simulink model "d_kundur1"  (Simulink 5.1)
settings: Solver=ode45  StartTime=0.0  StopTime=10.0  RelTol=1e-3
libraries: fm_lib x15
settings Model: Creator=fmilano  LastModifiedBy=fmilano  ExtModeAutoUpdateStatusClock=off  SignalLoggingName=logsout  BooleanDataType=on  RTWOptions="-aEnforceIntegerDowncast=1 -aFoldNonRolledExpr=1 -aInlineInvariantSignals=1 -aInlineParameters=0 -aLocalBlockOutputs=1 -aRollThreshold=5 -aZeroInternalMemoryAtStartup=1 -aZeroExternalMemoryAtStartup=1 -aInitFltsAndDblsToZero=1 -aForceBlockIOInitOptimize=0 -aGenerateReport=0 -aGenCodeOnly=0 -aRTWVerbose=1 -aIncludeHyperlinkInReport=0 -aLaunchReport=0 -aGenerateTraceInfo=0  -aForceParamTrailComments=0 -aGenerateComments=1 -aIgnoreCustomStorageClasses=1 -aIncHierarchyInIds=0 -aMaxRTWIdLen=31 -aShowEliminatedStatements=0 -aIncDataTypeInIds=0 -aInsertBlockDesc=0 -aIgnoreTestpoints=0 -aSimulinkBlockComments=1 -aInlinedPrmAccess=\"Literals\"  -aSuppressErrorStatus=0 -aModelReferenceCompliant=1 -aParenthesesLevel=\"Nominal\" -aModelStepFunctionPrototypeControlCompliant=0 -aPortableWordSizes=0 -aParMdlRefBuildCompliant=1 -aSupportNonInlinedSFcns=1 -aSupportContinuousTime=1 -aSupportComplex=1 -aSupportNonFinite=1 -aSupportAbsoluteTime=1 -aMultiwordLength=2048 -aTargetPreCompLibLocation=\"\" -aTargetLibSuffix=\"\" -aTargetFunctionLibrary=\"ANSI_C\" -aTargetFcnLib=\"ansi_tfl_tmw.mat\" -aMultiInstanceERTCode=0 -aLogVarNameModifier=\"rt_\" -aERTFirstTimeCompliant=0 -aIsPILTarget=0 -aCombineOutputUpdateFcns=0 -aGenerateASAP2=0 -aGenerateClassInterface=0 -aGenerateTestInterfaces=0 -aGenerateSampleERTMain=0 -aGenerateFullHeader=1 -aUtilityFuncGeneration=\"Auto\" -aIncludeFileDelimiter=\"Auto\" -aIncludeMdlTerminateFcn=1 -aPurelyIntegerCode=0 -aAutosarCompliant=0 -aERTCustomFileBanners=0 -aRTWCAPIStates=0 -aRTWCAPIParams=0 -aRTWCAPISignals=0 -aMatFileLogging=1 -aCompOptLevelCompliant=0 -aCPPClassGenCompliant=0 -aExtModeIntrfLevel=\"Level1\" -aExtModeMexFile=\"ext_comm\" -aExtModeTransport=0 -aExtModeStaticAllocSize=1000000 -aExtModeTesting=0 -aExtModeStaticAlloc=0 -aExtMode=0 -aERTMultiwordLength=256 -aERTMultiwordTypeDef=\"System defined\"  -aGenerateTraceInfo=0 -aGenerateTraceInfo=0 -aGenerateTraceInfo=0 -aGenerateTraceInfo=0 -aPrefixModelToSubsysFcnNames=1"

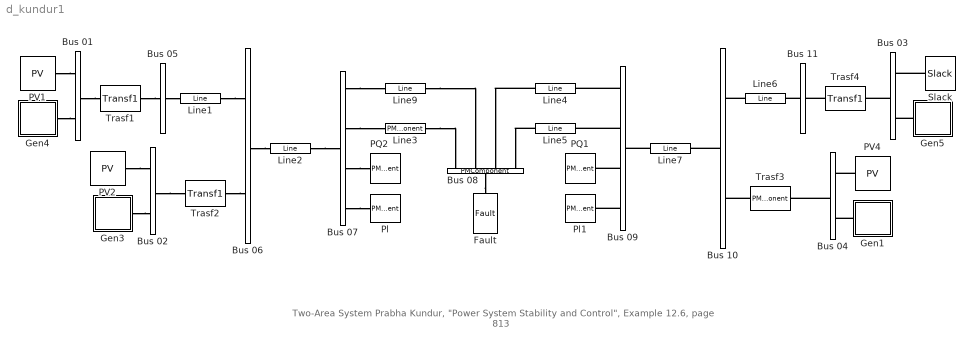
== system d_kundur1 ==
  note: Two-Area System
      | Prabha Kundur, "Power System Stability and Control", Example 12.6, page 813
  Bus 01 : PMComponent  Tag=PSATblock  Description=Connection  PhysicalDomain=psatdomain  LeftPortType=p1  RightPortType=p1  LConnTagsString=__newl0|__newl1  RConnTagsString=__newr0  mask(Bus){in=2, out=1, p2q=20, p3_4q=[1.03   0.3229], p5q=1, p6q=1}
      mask prompts: in "Number of inputs:"; out "Number of outputs:"; p2q "Voltage Rating [kV]"; p3_4q "Voltage initial guess [p.u.  rad]"; p5q "Area number"; p6q "Region number"
      mask help: Bus block.
      mask init:
      | fm_inout
      mask CallbackString: ||||fm_block|
      mask Display: plot([0 1 1 0 0],[0 0 1 1 0])
  Bus 02 : PMComponent  Tag=PSATblock  Description=Connection  PhysicalDomain=psatdomain  LeftPortType=p1  RightPortType=p1  LConnTagsString=__newl0|__newl1  RConnTagsString=__newr0  mask(Bus){in=2, out=1, p2q=20, p3_4q=[1.01   0.1536], p5q=1, p6q=1}
      mask prompts: in "Number of inputs:"; out "Number of outputs:"; p2q "Voltage Rating [kV]"; p3_4q "Voltage initial guess [p.u.  rad]"; p5q "Area number"; p6q "Region number"
      mask help: Bus block.
      mask init:
      | fm_inout
      mask CallbackString: ||||fm_block|
      mask Display: plot([0 1 1 0 0],[0 0 1 1 0])
  Bus 03 : PMComponent  Tag=PSATblock  Description=Connection  Orientation=left  PhysicalDomain=psatdomain  LeftPortType=p1  RightPortType=p1  LConnTagsString=__newl0|__newl1  RConnTagsString=__newr0  mask(Bus){in=2, out=1, p2q=20, p3_4q=[1.03  -0.1187], p5q=2, p6q=1}
      mask prompts: in "Number of inputs:"; out "Number of outputs:"; p2q "Voltage Rating [kV]"; p3_4q "Voltage initial guess [p.u.  rad]"; p5q "Area number"; p6q "Region number"
      mask help: Bus block.
      mask init:
      | fm_inout
      mask CallbackString: ||||fm_block|
      mask Display: plot([0 1 1 0 0],[0 0 1 1 0])
  Bus 04 : PMComponent  Tag=PSATblock  Description=Connection  Orientation=left  PhysicalDomain=psatdomain  LeftPortType=p1  RightPortType=p1  LConnTagsString=__newl0|__newl1  RConnTagsString=__newr0  mask(Bus){in=2, out=1, p2q=20, p3_4q=[1.01   -0.295], p5q=2, p6q=1}
      mask prompts: in "Number of inputs:"; out "Number of outputs:"; p2q "Voltage Rating [kV]"; p3_4q "Voltage initial guess [p.u.  rad]"; p5q "Area number"; p6q "Region number"
      mask help: Bus block.
      mask init:
      | fm_inout
      mask CallbackString: ||||fm_block|
      mask Display: plot([0 1 1 0 0],[0 0 1 1 0])
  Bus 05 : PMComponent  Tag=PSATblock  Description=Connection  PhysicalDomain=psatdomain  LeftPortType=p1  RightPortType=p1  LConnTagsString=__newl0  RConnTagsString=__newr0  mask(Bus){in=1, out=1, p2q=230, p3_4q=[1.01   0.2112], p5q=1, p6q=1}
      mask prompts: in "Number of inputs:"; out "Number of outputs:"; p2q "Voltage Rating [kV]"; p3_4q "Voltage initial guess [p.u.  rad]"; p5q "Area number"; p6q "Region number"
      mask help: Bus block.
      mask init:
      | fm_inout
      mask CallbackString: ||||fm_block|
      mask Display: plot([0 1 1 0 0],[0 0 1 1 0])
  Bus 06 : PMComponent  Tag=PSATblock  Description=Connection  PhysicalDomain=psatdomain  LeftPortType=p1  RightPortType=p1  LConnTagsString=__newl0|__newl1  RConnTagsString=__newr0  mask(Bus){in=2, out=1, p2q=230, p3_4q=[0.9876   0.03665], p5q=1, p6q=1}
      mask prompts: in "Number of inputs:"; out "Number of outputs:"; p2q "Voltage Rating [kV]"; p3_4q "Voltage initial guess [p.u.  rad]"; p5q "Area number"; p6q "Region number"
      mask help: Bus block.
      mask init:
      | fm_inout
      mask CallbackString: ||||fm_block|
      mask Display: plot([0 1 1 0 0],[0 0 1 1 0])
  Bus 07 : PMComponent  Tag=PSATblock  Description=Connection  PhysicalDomain=psatdomain  LeftPortType=p1  RightPortType=p1  LConnTagsString=__newl0  RConnTagsString=__newr0|__newr1|__newr2|__newr3  mask(Bus){in=1, out=4, p2q=230, p3_4q=[1   -0.1065], p5q=1, p6q=1}
      mask prompts: in "Number of inputs:"; out "Number of outputs:"; p2q "Voltage Rating [kV]"; p3_4q "Voltage initial guess [p.u.  rad]"; p5q "Area number"; p6q "Region number"
      mask help: Bus block.
      mask init:
      | fm_inout
      mask CallbackString: ||||fm_block|
      mask Display: plot([0 1 1 0 0],[0 0 1 1 0])
  Bus 08 : PMComponent  Tag=PSATblock  Description=Connection  Orientation=down  PhysicalDomain=psatdomain  LeftPortType=p1  RightPortType=p1  LConnTagsString=__newl0|__newl1|__newl2|__newl3  RConnTagsString=__newr0  mask(Bus){in=4, out=1, p2q=230, p3_4q=[1.0   -0.3368], p5q=3, p6q=1}
      mask prompts: in "Number of inputs:"; out "Number of outputs:"; p2q "Voltage Rating [kV]"; p3_4q "Voltage initial guess [p.u.  rad]"; p5q "Area number"; p6q "Region number"
      mask help: Bus block.
      mask init:
      | fm_inout
      mask CallbackString: ||||fm_block|
      mask Display: plot([0 1 1 0 0],[0 0 1 1 0])
  Bus 09 : PMComponent  Tag=PSATblock  Description=Connection  Orientation=left  PhysicalDomain=psatdomain  LeftPortType=p1  RightPortType=p1  LConnTagsString=__newl0  RConnTagsString=__newr0|__newr1|__newr2|__newr3  mask(Bus){in=1, out=4, p2q=230, p3_4q=[0.9899   -0.555], p5q=2, p6q=1}
      mask prompts: in "Number of inputs:"; out "Number of outputs:"; p2q "Voltage Rating [kV]"; p3_4q "Voltage initial guess [p.u.  rad]"; p5q "Area number"; p6q "Region number"
      mask help: Bus block.
      mask init:
      | fm_inout
      mask CallbackString: ||||fm_block|
      mask Display: plot([0 1 1 0 0],[0 0 1 1 0])
  Bus 10 : PMComponent  Tag=PSATblock  Description=Connection  Orientation=left  PhysicalDomain=psatdomain  LeftPortType=p1  RightPortType=p1  LConnTagsString=__newl0|__newl1  RConnTagsString=__newr0  mask(Bus){in=2, out=1, p2q=230, p3_4q=[0.9938   -0.4119], p5q=2, p6q=1}
      mask prompts: in "Number of inputs:"; out "Number of outputs:"; p2q "Voltage Rating [kV]"; p3_4q "Voltage initial guess [p.u.  rad]"; p5q "Area number"; p6q "Region number"
      mask help: Bus block.
      mask init:
      | fm_inout
      mask CallbackString: ||||fm_block|
      mask Display: plot([0 1 1 0 0],[0 0 1 1 0])
  Bus 11 : PMComponent  Tag=PSATblock  Description=Connection  Orientation=left  PhysicalDomain=psatdomain  LeftPortType=p1  RightPortType=p1  LConnTagsString=__newl0  RConnTagsString=__newr0  mask(Bus){in=1, out=1, p2q=230, p3_4q=[1.013   -0.233900], p5q=2, p6q=1}
      mask prompts: in "Number of inputs:"; out "Number of outputs:"; p2q "Voltage Rating [kV]"; p3_4q "Voltage initial guess [p.u.  rad]"; p5q "Area number"; p6q "Region number"
      mask help: Bus block.
      mask init:
      | fm_inout
      mask CallbackString: ||||fm_block|
      mask Display: plot([0 1 1 0 0],[0 0 1 1 0])
  Fault : fm_lib/Faults &  Breakers/Fault  Tag=PSATblock  Description=Faults & Breakers  Orientation=down  PhysicalDomain=psatdomain  SubClassName=unknown  LeftPortType=p1  RightPortType=p1  LConnTagsString=__newl0  p2_3_4q="[100  230  60]"  p5q=1  p6q=1.050  p7q=0  p8q=1e-5
  Gen1 : Subsystem  Tag=PSATblock  Description=Machines  Orientation=left  mask(Syn){p2_3_4q=[900  20  60], p5q=6, p7_6q=[0.0025  0.2], p8_9_10q=[1.80  0.30  0.25], p11_12q=[8.00  0.03], p13_14_15q=[1.70  0.55  0.25], p16_17q=[0.4  0.05], p18_19q=[12.35  0.00], p20_21q=[0.00  0.00], p22_23q=[1.00  1.00], p24q=0.0, p25_26q=[0 0], in=0, p27q=1, p28q=on}
      mask prompts: p2_3_4q "Power, voltage and frequency ratings [MVA, kV, Hz]"; p5q "Machine Dynamic Order"; p7_6q "resistance ra and leakage reactance xl [p.u. p.u.]"; p8_9_10q "d-axis reactances Xd, X'd X"d [p.u.,p.u.,p.u.]"; p11_12q "d-axis open circuit time constants T'd0 and T"d0 [s, s]"; p13_14_15q "q-axis reactances Xq, X'q, X"q [p.u.  p.u.  p.u.]"; p16_17q "q-axis open circuit time constants T'q0 and T"q0 [s s]"; p18_19q "Inertia (M = 2H) and Damping [s, p.u.]"; p20_21q "Speed and active power additional signals Kw and Kp [p.u., p.u.]"; p22_23q "Percentage of active and reactive powers at bus [p.u. p.u.]"; p24q "d-axis additional circuit leakage time constant Taa [s]"; p25_26q "Saturation coefficients S(1.0) and S(1.2)"; in "Number of input signals"; p27q "COI number"; p28q "Connected"
      mask help: This block defines a fourth order synchronous machine.
      mask init:
      | fm_inout
      | [x,y] = fm_draw('circle');
      | [xg,yg] = fm_draw('G');
      | [xs,ys] = fm_draw('sinus');
      mask StyleString: edit,popup(8|6|5.3|5.2|5.1|4|3|2),edit,edit,edit,edit,edit,edit,edit,edit,edit,edit,popup(0|1|2),edit,checkbox
      mask CallbackString: |fm_block|||||||||||||fm_block
      mask Display:
      | plot(x+1.4,y,0.12*xs+1,0.15*ys-0.6)
      | color('blue')
      | plot(1.4+0.45*xg,0.3+0.45*yg)
  Gen3 : Subsystem  Tag=PSATblock  Description=Machines  mask(Syn){p2_3_4q=[900  20  60], p5q=6, p7_6q=[0.0025  0.2], p8_9_10q=[1.80  0.30  0.25], p11_12q=[8.00  0.03], p13_14_15q=[1.70  0.55  0.25], p16_17q=[0.4  0.05], p18_19q=[13.00  0.00], p20_21q=[0.00  0.00], p22_23q=[1.00  1.00], p24q=0.0, p25_26q=[0 0], in=0, p27q=1, p28q=on}
      mask prompts: p2_3_4q "Power, voltage and frequency ratings [MVA, kV, Hz]"; p5q "Machine Dynamic Order"; p7_6q "resistance ra and leakage reactance xl [p.u. p.u.]"; p8_9_10q "d-axis reactances Xd, X'd X"d [p.u.,p.u.,p.u.]"; p11_12q "d-axis open circuit time constants T'd0 and T"d0 [s, s]"; p13_14_15q "q-axis reactances Xq, X'q, X"q [p.u.  p.u.  p.u.]"; p16_17q "q-axis open circuit time constants T'q0 and T"q0 [s s]"; p18_19q "Inertia (M = 2H) and Damping [s, p.u.]"; p20_21q "Speed and active power additional signals Kw and Kp [p.u., p.u.]"; p22_23q "Percentage of active and reactive powers at bus [p.u. p.u.]"; p24q "d-axis additional circuit leakage time constant Taa [s]"; p25_26q "Saturation coefficients S(1.0) and S(1.2)"; in "Number of input signals"; p27q "COI number"; p28q "Connected"
      mask help: This block defines a fourth order synchronous machine.
      mask init:
      | fm_inout
      | [x,y] = fm_draw('circle');
      | [xg,yg] = fm_draw('G');
      | [xs,ys] = fm_draw('sinus');
      mask StyleString: edit,popup(8|6|5.3|5.2|5.1|4|3|2),edit,edit,edit,edit,edit,edit,edit,edit,edit,edit,popup(0|1|2),edit,checkbox
      mask CallbackString: |fm_block|||||||||||||fm_block
      mask Display:
      | plot(x+1.4,y,0.12*xs+1,0.15*ys-0.6)
      | color('blue')
      | plot(1.4+0.45*xg,0.3+0.45*yg)
  Gen4 : Subsystem  Tag=PSATblock  Description=Machines  mask(Syn){p2_3_4q=[900  20  60], p5q=6, p7_6q=[0.0025  0.2], p8_9_10q=[1.80  0.30  0.25], p11_12q=[8.00  0.03], p13_14_15q=[1.70  0.55  0.25], p16_17q=[0.4  0.05], p18_19q=[13.00  0.00], p20_21q=[0.00  0.00], p22_23q=[1.00  1.00], p24q=0.002, p25_26q=[0 0], in=0, p27q=1, p28q=on}
      mask prompts: p2_3_4q "Power, voltage and frequency ratings [MVA, kV, Hz]"; p5q "Machine Dynamic Order"; p7_6q "resistance ra and leakage reactance xl [p.u. p.u.]"; p8_9_10q "d-axis reactances Xd, X'd X"d [p.u.,p.u.,p.u.]"; p11_12q "d-axis open circuit time constants T'd0 and T"d0 [s, s]"; p13_14_15q "q-axis reactances Xq, X'q, X"q [p.u.  p.u.  p.u.]"; p16_17q "q-axis open circuit time constants T'q0 and T"q0 [s s]"; p18_19q "Inertia (M = 2H) and Damping [s, p.u.]"; p20_21q "Speed and active power additional signals Kw and Kp [p.u., p.u.]"; p22_23q "Percentage of active and reactive powers at bus [p.u. p.u.]"; p24q "d-axis additional circuit leakage time constant Taa [s]"; p25_26q "Saturation coefficients S(1.0) and S(1.2)"; in "Number of input signals"; p27q "COI number"; p28q "Connected"
      mask help: This block defines a fourth order synchronous machine.
      mask init:
      | fm_inout
      | [x,y] = fm_draw('circle');
      | [xg,yg] = fm_draw('G');
      | [xs,ys] = fm_draw('sinus');
      mask StyleString: edit,popup(8|6|5.3|5.2|5.1|4|3|2),edit,edit,edit,edit,edit,edit,edit,edit,edit,edit,popup(0|1|2),edit,checkbox
      mask CallbackString: |fm_block|||||||||||||fm_block
      mask Display:
      | plot(x+1.4,y,0.12*xs+1,0.15*ys-0.6)
      | color('blue')
      | plot(1.4+0.45*xg,0.3+0.45*yg)
  Gen5 : Subsystem  Tag=PSATblock  Description=Machines  Orientation=left  mask(Syn){p2_3_4q=[900  20  60], p5q=6, p7_6q=[0.0025  0.2], p8_9_10q=[1.80  0.30  0.25], p11_12q=[8.00  0.03], p13_14_15q=[1.70  0.55  0.25], p16_17q=[0.4  0.05], p18_19q=[12.35  0.00], p20_21q=[0.00  0.00], p22_23q=[1.00  1.00], p24q=0.0, p25_26q=[0 0], in=0, p27q=1, p28q=on}
      mask prompts: p2_3_4q "Power, voltage and frequency ratings [MVA, kV, Hz]"; p5q "Machine Dynamic Order"; p7_6q "resistance ra and leakage reactance xl [p.u. p.u.]"; p8_9_10q "d-axis reactances Xd, X'd X"d [p.u.,p.u.,p.u.]"; p11_12q "d-axis open circuit time constants T'd0 and T"d0 [s, s]"; p13_14_15q "q-axis reactances Xq, X'q, X"q [p.u.  p.u.  p.u.]"; p16_17q "q-axis open circuit time constants T'q0 and T"q0 [s s]"; p18_19q "Inertia (M = 2H) and Damping [s, p.u.]"; p20_21q "Speed and active power additional signals Kw and Kp [p.u., p.u.]"; p22_23q "Percentage of active and reactive powers at bus [p.u. p.u.]"; p24q "d-axis additional circuit leakage time constant Taa [s]"; p25_26q "Saturation coefficients S(1.0) and S(1.2)"; in "Number of input signals"; p27q "COI number"; p28q "Connected"
      mask help: This block defines a fourth order synchronous machine.
      mask init:
      | fm_inout
      | [x,y] = fm_draw('circle');
      | [xg,yg] = fm_draw('G');
      | [xs,ys] = fm_draw('sinus');
      mask StyleString: edit,popup(8|6|5.3|5.2|5.1|4|3|2),edit,edit,edit,edit,edit,edit,edit,edit,edit,edit,popup(0|1|2),edit,checkbox
      mask CallbackString: |fm_block|||||||||||||fm_block
      mask Display:
      | plot(x+1.4,y,0.12*xs+1,0.15*ys-0.6)
      | color('blue')
      | plot(1.4+0.45*xg,0.3+0.45*yg)
  Line1 : fm_lib/Power Flow/Line  Tag=PSATblock  Description=Power Flow  PhysicalDomain=psatdomain  SubClassName=unknown  LeftPortType=p1  RightPortType=p1  LConnTagsString=__newl0  RConnTagsString=__newr0  p3_4_5q="[100  230  60]"  p6q=0  p8q=0.0001*25  p9q=0.001*25  p10q=0.00175*25  p13_14_15q="[1.0  0.0  0.0]"  p16q=on
  Line2 : fm_lib/Power Flow/Line  Tag=PSATblock  Description=Power Flow  PhysicalDomain=psatdomain  SubClassName=unknown  LeftPortType=p1  RightPortType=p1  LConnTagsString=__newl0  RConnTagsString=__newr0  p3_4_5q="[100  230  60]"  p6q=0  p8q=0.0001*10  p9q=0.001*10  p10q=0.00175*10  p13_14_15q="[1.0  0.0  0.0]"  p16q=on
  Line3 : PMComponent  Tag=PSATblock  Description=Power Flow  PhysicalDomain=psatdomain  LeftPortType=p1  RightPortType=p1  LConnTagsString=__newl0  RConnTagsString=__newr0  mask(Line){p3_4_5q=[100  230  60], p6q=0, p8q=0.0001*110, p9q=0.001*110, p10q=0.00175*110, p13_14_15q=[1.0  0.0  0.0], p16q=on}
      mask prompts: p3_4_5q "Power, Voltage and Frequency Ratings [MVA, kV, Hz]"; p6q "Length of line [km] (0 for p.u. parameters)"; p8q "Resistance [p.u. (Ohms/km)]"; p9q "Reactance [p.u. (H/km)]"; p10q "Susceptance [p.u. (F/km)]"; p13_14_15q "Imax, Pmax and Smax [p.u., p.u., p.u.]"; p16q "Connected"
      mask help: This block defines a pi model for a tree phase line.
      mask init:
      | [xp,yp] = fm_draw('pi');
      mask CallbackString: ||||||fm_block
      mask Display:
      | plot([-1  1  1 -1 -1],[-0.2 -0.2 0.2 0.2 -0.2])
      | color('blue')
      | plot(0.35*xp,0.2*yp)
  Line4 : fm_lib/Power Flow/Line  Tag=PSATblock  Description=Power Flow  PhysicalDomain=psatdomain  SubClassName=unknown  LeftPortType=p1  RightPortType=p1  LConnTagsString=__newl0  RConnTagsString=__newr0  p3_4_5q="[100  230  60]"  p6q=0  p8q=0.0001*110  p9q=0.001*110  p10q=0.00175*110/2  p13_14_15q="[1.0  0.0  0.0]"  p16q=on
  Line5 : fm_lib/Power Flow/Line  Tag=PSATblock  Description=Power Flow  PhysicalDomain=psatdomain  SubClassName=unknown  LeftPortType=p1  RightPortType=p1  LConnTagsString=__newl0  RConnTagsString=__newr0  p3_4_5q="[100  230  60]"  p6q=0  p8q=0.0001*110  p9q=0.001*110  p10q=0.00175*110  p13_14_15q="[1.0  0.0  0.0]"  p16q=on
  Line6 : fm_lib/Power Flow/Line  Tag=PSATblock  Description=Power Flow  Orientation=left  PhysicalDomain=psatdomain  SubClassName=unknown  LeftPortType=p1  RightPortType=p1  LConnTagsString=__newl0  RConnTagsString=__newr0  p3_4_5q="[100  230  60]"  p6q=0  p8q=0.0001*25  p9q=0.001*25  p10q=0.00175*25  p13_14_15q="[1.0  0.0  0.0]"  p16q=on
  Line7 : fm_lib/Power Flow/Line  Tag=PSATblock  Description=Power Flow  PhysicalDomain=psatdomain  SubClassName=unknown  LeftPortType=p1  RightPortType=p1  LConnTagsString=__newl0  RConnTagsString=__newr0  p3_4_5q="[100  230  60]"  p6q=0  p8q=0.0001*10  p9q=0.001*10  p10q=0.00175*10  p13_14_15q="[1.0  0.0  0.0]"  p16q=on
  Line9 : fm_lib/Power Flow/Line  Tag=PSATblock  Description=Power Flow  PhysicalDomain=psatdomain  SubClassName=unknown  LeftPortType=p1  RightPortType=p1  LConnTagsString=__newl0  RConnTagsString=__newr0  p3_4_5q="[100  230  60]"  p6q=0  p8q=0.0001*110  p9q=0.001*110  p10q=0.00175*110/2  p13_14_15q="[1.0  0.0  0.0]"  p16q=on
  PQ1 : PMComponent  Tag=PSATblock  Description=Power Flow  Orientation=left  PhysicalDomain=psatdomain  LeftPortType=p1  RightPortType=p1  LConnTagsString=__newl0  mask(PQ){p2_3q=[100  230], p4_5q=[17.67  -2.5], p6_7q=[1.05  0.95], p8q=off}
      mask prompts: p2_3q "Power and Voltage Ratings [MVA, kV]"; p4_5q "Active and Reactive Powers [p.u.  p.u.]"; p6_7q "Maximum and Minimum Allowable Voltage [p.u.   p.u.]"; p8q "Allow conversion to impendance for min & max voltage"
      mask help:
      | This block defines a constant power load:
      |
      | P = Pcost.
      | Q = Qcost.
      mask CallbackString: |||fm_block
      mask Display: plot([1 -0.5 -0.5 1],[0 0.866 -0.866 0])
  PQ2 : PMComponent  Tag=PSATblock  Description=Power Flow  PhysicalDomain=psatdomain  LeftPortType=p1  RightPortType=p1  LConnTagsString=__newl0  mask(PQ){p2_3q=[100  230], p4_5q=[9.67  -1], p6_7q=[1.05  0.95], p8q=off}
      mask prompts: p2_3q "Power and Voltage Ratings [MVA, kV]"; p4_5q "Active and Reactive Powers [p.u.  p.u.]"; p6_7q "Maximum and Minimum Allowable Voltage [p.u.   p.u.]"; p8q "Allow conversion to impendance for min & max voltage"
      mask help:
      | This block defines a constant power load:
      |
      | P = Pcost.
      | Q = Qcost.
      mask CallbackString: |||fm_block
      mask Display: plot([1 -0.5 -0.5 1],[0 0.866 -0.866 0])
  PV1 : fm_lib/Power Flow/PV  Tag=PSATblock  Description=Power Flow  PhysicalDomain=psatdomain  SubClassName=unknown  LeftPortType=p1  RightPortType=p1  RConnTagsString=__newr0  p2_3q="[100  20]"  p4q=7  p5q=1.03  p6_7q=[5 -2]  p8_9q="[1.1  0.9]"  p10q=1  p11q=on
  PV2 : fm_lib/Power Flow/PV  Tag=PSATblock  Description=Power Flow  PhysicalDomain=psatdomain  SubClassName=unknown  LeftPortType=p1  RightPortType=p1  RConnTagsString=__newr0  p2_3q="[100  20]"  p4q=7  p5q=1.01  p6_7q=[5 -2]  p8_9q="[1.1  0.9]"  p10q=1  p11q=on
  PV4 : fm_lib/Power Flow/PV  Tag=PSATblock  Description=Power Flow  Orientation=left  PhysicalDomain=psatdomain  SubClassName=unknown  LeftPortType=p1  RightPortType=p1  RConnTagsString=__newr0  p2_3q="[100  20]"  p4q=7  p5q=1.01  p6_7q=[5 -2]  p8_9q="[1.1  0.9]"  p10q=1  p11q=on
  Pl : PMComponent  Tag=PSATblock  Description=Loads  PhysicalDomain=psatdomain  LeftPortType=p1  RightPortType=p1  LConnTagsString=__newl0  mask(Pl){p2_3_4q=[100 230 60], p5_6_7q=[0 100 0], p8_9_10q=[0 0 100], p11q=on, p12q=on}
      mask prompts: p2_3_4q "Power, voltage and frequency ratings [MVA, kV, Hz]"; p5_6_7q "Percentage of resistance, active current and active power [%, %, %]"; p8_9_10q "Percentage of reactance, reactive current and reactive power [%, %, %]"; p11q "Initialize after power flow"; p12q "Connected"
      mask help: This block defines a ZIP load.
      mask CallbackString: |||fm_block|fm_block
      mask Display:
      | plot([-1 -1 1 1 -1],[-1 1 1 -1 -1])
      | color('blue')
      | plot([0 0],[-0.3 0.3],[-0.3 -0.7 -0.3 -0.7],[-0.3 -0.3 0.3 0.3])
      | plot([0.3 0.3 0.6 0.7 0.7 0.6 0.3],[-0.3 0.3 0.3 0.2 0.1 0 0])
  Pl1 : PMComponent  Tag=PSATblock  Description=Loads  Orientation=left  PhysicalDomain=psatdomain  LeftPortType=p1  RightPortType=p1  LConnTagsString=__newl0  mask(Pl){p2_3_4q=[100 230 60], p5_6_7q=[0 100 0], p8_9_10q=[0 0 100], p11q=on, p12q=on}
      mask prompts: p2_3_4q "Power, voltage and frequency ratings [MVA, kV, Hz]"; p5_6_7q "Percentage of resistance, active current and active power [%, %, %]"; p8_9_10q "Percentage of reactance, reactive current and reactive power [%, %, %]"; p11q "Initialize after power flow"; p12q "Connected"
      mask help: This block defines a ZIP load.
      mask CallbackString: |||fm_block|fm_block
      mask Display:
      | plot([-1 -1 1 1 -1],[-1 1 1 -1 -1])
      | color('blue')
      | plot([0 0],[-0.3 0.3],[-0.3 -0.7 -0.3 -0.7],[-0.3 -0.3 0.3 0.3])
      | plot([0.3 0.3 0.6 0.7 0.7 0.6 0.3],[-0.3 0.3 0.3 0.2 0.1 0 0])
  Slack : fm_lib/Power Flow/Slack  Tag=PSATblock  Description=Power Flow  Orientation=left  PhysicalDomain=psatdomain  SubClassName=unknown  LeftPortType=p1  RightPortType=p1  RConnTagsString=__newr0  p2_3q="[100  20]"  p4q=1.03  p5q=- 0.118682389135614  p6_7q=[99 -99]  p8_9q="[1.1  0.9]"  p10q=7  p11q=1  p12q=on  p13q=on
  Trasf1 : fm_lib/Power Flow/Transf1  Tag=PSATblock  Description=Power Flow  PhysicalDomain=psatdomain  SubClassName=unknown  LeftPortType=p1  RightPortType=p1  LConnTagsString=__newl0  RConnTagsString=__newr0  p3_4_5q="[900  20 60]"  p7q=20/230  p8q=0.0  p9q=0.15  p13_14_15q="[1.0  0.0  0.0]"  p16q=on
  Trasf2 : fm_lib/Power Flow/Transf1  Tag=PSATblock  Description=Power Flow  PhysicalDomain=psatdomain  SubClassName=unknown  LeftPortType=p1  RightPortType=p1  LConnTagsString=__newl0  RConnTagsString=__newr0  p3_4_5q="[900  20 60]"  p7q=20/230  p8q=0.0  p9q=0.15  p13_14_15q="[1.0  0.0  0.0]"  p16q=on
  Trasf3 : PMComponent  Tag=PSATblock  Description=Power Flow  Orientation=left  PhysicalDomain=psatdomain  LeftPortType=p1  RightPortType=p1  LConnTagsString=__newl0  RConnTagsString=__newr0  mask(Line){p3_4_5q=[900  20 60], p7q=20/230, p8q=0.0, p9q=0.15, p13_14_15q=[1.0  0.0  0.0], p16q=on}
      mask prompts: p3_4_5q "Power, Voltage and Frequency Ratings [MVA, kV, Hz]"; p7q "Primary and secondary voltage ratio [kV/kV]"; p8q "Resistance [p.u.]"; p9q "Reactance [p.u.]"; p13_14_15q "Imax, Pmax and Smax [p.u., p.u., p.u.]"; p16q "Connected"
      mask help: This block defines a transformer.
      mask init:
      | [x,y] = fm_draw('circle');
      | [x1,y1] = fm_draw('1');
      | [x2,y2] = fm_draw('2');
      mask CallbackString: |||||fm_block
      mask Display:
      | plot(x,y,x+1.4,y,[-1 -1.3],[0 0],[2.4 2.7],[0 0])
      | color('green')
      | plot(-0.1+0.65*x1,0.65*y1)
      | plot(1.5+0.65*x2,0.65*y2)
  Trasf4 : fm_lib/Power Flow/Transf1  Tag=PSATblock  Description=Power Flow  Orientation=left  PhysicalDomain=psatdomain  SubClassName=unknown  LeftPortType=p1  RightPortType=p1  LConnTagsString=__newl0  RConnTagsString=__newr0  p3_4_5q="[900  20 60]"  p7q=20/230  p8q=0.0  p9q=0.15  p13_14_15q="[1.0  0.0  0.0]"  p16q=on
  connections:
  Line3/RConn1 -- Bus 08/LConn1
  Line9/RConn1 -- Bus 08/LConn2
  Bus 09/RConn4 -- Pl1/LConn1
  Bus 07/RConn4 -- Pl/LConn1
  Line5/LConn1 -- Bus 08/LConn4
  Line4/LConn1 -- Bus 08/LConn3
  Line2/RConn1 -- Bus 07/LConn1
  Bus 07/RConn3 -- PQ2/LConn1
  Bus 09/RConn3 -- PQ1/LConn1
  Bus 09/RConn2 -- Line5/RConn1
  Bus 09/RConn1 -- Line4/RConn1
  Line7/LConn1 -- Bus 09/LConn1
  Bus 10/RConn1 -- Line7/RConn1
  Trasf3/RConn1 -- Bus 10/LConn2
  Line6/RConn1 -- Bus 10/LConn1
  Bus 04/RConn1 -- Trasf3/LConn1
  Gen1/RConn1 -- Bus 04/LConn2
  PV4/RConn1 -- Bus 04/LConn1
  Bus 11/RConn1 -- Line6/LConn1
  Trasf4/RConn1 -- Bus 11/LConn1
  Bus 03/RConn1 -- Trasf4/LConn1
  Gen5/RConn1 -- Bus 03/LConn2
  Slack/RConn1 -- Bus 03/LConn1
  Bus 06/RConn1 -- Line2/LConn1
  Trasf2/RConn1 -- Bus 06/LConn2
  Bus 02/RConn1 -- Trasf2/LConn1
  Gen3/RConn1 -- Bus 02/LConn2
  PV2/RConn1 -- Bus 02/LConn1
  Line1/RConn1 -- Bus 06/LConn1
  Bus 07/RConn2 -- Line3/LConn1
  Bus 07/RConn1 -- Line9/LConn1
  Bus 05/RConn1 -- Line1/LConn1
  Bus 01/RConn1 -- Trasf1/LConn1
  Trasf1/RConn1 -- Bus 05/LConn1
  Gen4/RConn1 -- Bus 01/LConn2
  PV1/RConn1 -- Bus 01/LConn1
  Bus 08/RConn1 -- Fault/LConn1

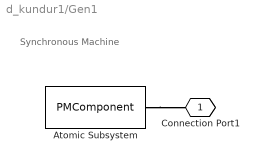
== system d_kundur1/Gen1 ==
  note: Synchronous Machine
  Atomic Subsystem : PMComponent  PhysicalDomain=psatdomain  LeftPortType=p1  RightPortType=p1  RConnTagsString=__newr0
  Connection Port1 : PMIOPort  Tag=PMCPort  Orientation=left  Port=1  Side=Right
  connections:
  Atomic Subsystem/RConn1 -- Connection Port1/RConn1

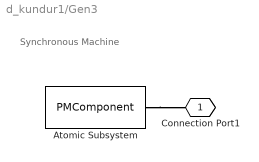
== system d_kundur1/Gen3 ==
  note: Synchronous Machine
  Atomic Subsystem : PMComponent  PhysicalDomain=psatdomain  LeftPortType=p1  RightPortType=p1  RConnTagsString=__newr0
  Connection Port1 : PMIOPort  Tag=PMCPort  Orientation=left  Port=1  Side=Right
  connections:
  Atomic Subsystem/RConn1 -- Connection Port1/RConn1

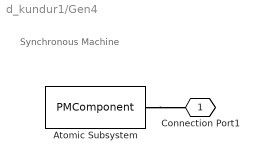
== system d_kundur1/Gen4 ==
  note: Synchronous Machine
  Atomic Subsystem : PMComponent  PhysicalDomain=psatdomain  LeftPortType=p1  RightPortType=p1  RConnTagsString=__newr0
  Connection Port1 : PMIOPort  Tag=PMCPort  Orientation=left  Port=1  Side=Right
  connections:
  Atomic Subsystem/RConn1 -- Connection Port1/RConn1

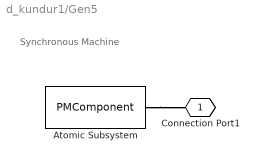
== system d_kundur1/Gen5 ==
  note: Synchronous Machine
  Atomic Subsystem : PMComponent  PhysicalDomain=psatdomain  LeftPortType=p1  RightPortType=p1  RConnTagsString=__newr0
  Connection Port1 : PMIOPort  Tag=PMCPort  Orientation=left  Port=1  Side=Right
  connections:
  Atomic Subsystem/RConn1 -- Connection Port1/RConn1
